simulink library "adi_ad9361_models_org"  (Simulink 10.0)
settings: Solver=VariableStepAuto  StartTime=0.0  StopTime=10.0  RelTol=1e-3
undefined symbols (not defined in the file): ad9361_preload, D, dBval, DCLeak_Matrix, designMultirateFIR, errordlg, fuzz_val, GainImb_Matrix, IP2_Matrix, IP3_Matrix, magnitude
libraries: simrfV2elements x20, simrfV2util1 x10, dsparch4 x8, simrfV2junction1 x8, simulink x8, dspmlti4 x6, ad9361_private x4, simulink_extras x2, dspsigattribs x2, simrfV2sources1 x2, simrfV2_lib x2, dspmathops x2
(part 2 of 2)

== system adi_ad9361_models_org/ad9361_rx/RF_RX/External LNA ==
  ExternalLNA on/off : Inport
  Amplifier : simrfV2elements/Amplifier  classname=amplifier  DataSource=Data file  File=unitygain.s2p  Paramtype=S-parameters  Sparam=[0 0;1 0]  SparamFreq=1e9 Hz  SparamZ0=50  Residues=0  Poles=0  DF={0 0; 1 0}  Source_linear_gain=Available power gain  linear_gain=0 dB  Zin=50  Zout=50  Source_Poly=Even and odd order  Poly_Coeffs=[0 1]  IPType=Output  IP2=inf dBm  IP3=inf dBm  P1dB=inf dBm  Psat=inf dBm  Gcomp=inf dBm  InternalGrounding=on  SourceFreq=Extracted from data source  PlotFreq=[1e9:1e6:3e9] Hz  PlotType=X-Y plane  YParam1=S11  YFormat1=Magnitude (decibels)  YParam2=None  YFormat2=Magnitude (decibels)  YOption=Linear  XOption=Linear  SparamRepresentation=Time domain (rationalfit)  FitTol=-40  FitOpt=Fit individually  AutoImpulseLength=on  ImpulseLength=1e-10 s  MagModeling=off  AddNoise=on  NoiseType=Noise figure  NoiseDist=White  NF=0  MinNF=0  Gopt=0  RN=0  CarrierFreq=0 Hz  NoiseAutoImpulseLength=on  NoiseImpulseLength=1e-10 s  SpecifyOpFreq=off  OpFreq=0 Hz
      settings: SourceProductName=RF Blockset  SourceProductBaseCode=RB
  Bypass : simrfV2junction1/Switch  classname=switch  Ron=0 Ohm  Roff=inf Ohm  Vthres=0.5 V
      settings: SourceProductName=RF Blockset  SourceProductBaseCode=RB
  Invert Control : Subsystem
  LNA on input : simrfV2junction1/Switch  classname=switch  Ron=0 Ohm  Roff=inf Ohm  Vthres=0.5 V
      settings: SourceProductName=RF Blockset  SourceProductBaseCode=RB
  LNA on ouput : simrfV2junction1/Switch  classname=switch  Ron=0 Ohm  Roff=inf Ohm  Vthres=0.5 V
      settings: SourceProductName=RF Blockset  SourceProductBaseCode=RB
  in : PMIOPort  Side=Left
  out : PMIOPort  Port=2  Side=Right
  wires:
  Invert Control/1(Out) -> Bypass/1
  ExternalLNA on/off/1 -> Invert Control/1(In), LNA on input/1, LNA on ouput/1
  connections:
  Amplifier/RConn1 -- LNA on ouput/LConn1
  Amplifier/LConn1 -- LNA on input/RConn1
  in/RConn1 -- Bypass/LConn1 -- LNA on input/LConn1
  LNA on ouput/RConn1 -- out/RConn1 -- Bypass/RConn1

== system adi_ad9361_models_org/ad9361_rx/RF_RX/RF Non Idealities ==
  LPF : Inport
  TIA : Inport  Port=2
  Demod : Inport  Port=3
  LNA : Inport  Port=4
  DetectChange : Subsystem
  RF Non Idealities : Subsystem
  DCLeakage : Outport  VectorParamsAs1DForOutWhenUnconnected=off
  GainImbalance : Outport  Port=2  VectorParamsAs1DForOutWhenUnconnected=off
  IP2 : Outport  Port=3  VectorParamsAs1DForOutWhenUnconnected=off
  IP3 : Outport  Port=4  VectorParamsAs1DForOutWhenUnconnected=off
  wires:
  DetectChange/1(Trigger) -> RF Non Idealities/Trigger
  RF Non Idealities/4(IP3) -> IP3/1
  RF Non Idealities/3(IP2) -> IP2/1
  RF Non Idealities/2(GainImbalance) -> GainImbalance/1
  RF Non Idealities/1(DCLeakage) -> DCLeakage/1
  LNA/1 -> DetectChange/1(In1), RF Non Idealities/1(LNA)
  Demod/1 -> DetectChange/2(In2), RF Non Idealities/2(Demod)
  LPF/1 -> DetectChange/4(In4), RF Non Idealities/4(LPF)
  TIA/1 -> DetectChange/3(In3), RF Non Idealities/3(TIA)

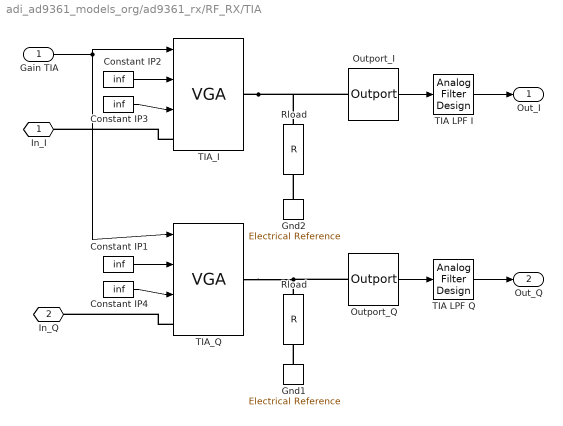
== system adi_ad9361_models_org/ad9361_rx/RF_RX/TIA ==
  Gain TIA : Inport
  " Rload" : simrfV2elements/R  classname=resistor  Resistance=100 Ohm  AddNoise=on
      settings: SourceProductName=RF Blockset  SourceProductBaseCode=RB
  Constant IP{1..4} (4 alike) : Constant  Value=inf
  Gnd1 : simrfV2_lib/Elements/Electrical Reference
      settings: SourceProductName=RF Blockset  SourceProductBaseCode=RB  InternalSimscapePortConfiguration="{\"Bottom\":[],\"Left\":[{\"id\":\"V\",\"label\":\"\",\"type\":\"foundation.rf.circuitenvelope\"}],\"Right\":[],\"Top\":[]}"
  Gnd2 : simrfV2_lib/Elements/Electrical Reference
      settings: SourceProductName=RF Blockset  SourceProductBaseCode=RB  InternalSimscapePortConfiguration="{\"Bottom\":[],\"Left\":[{\"id\":\"V\",\"label\":\"\",\"type\":\"foundation.rf.circuitenvelope\"}],\"Right\":[],\"Top\":[]}"
  Outport_I : simrfV2util1/Outport  SensorType=Ideal voltage  OutputFormat=Real Passband  CarrierFreq=abs(RF-LO) Hz  ZL=Inf  InternalGrounding=on  StepSize=Tstep s  AutoStep=off
      settings: SourceProductName=RF Blockset  SourceProductBaseCode=RB
  Outport_Q : simrfV2util1/Outport  SensorType=Ideal voltage  OutputFormat=Real Passband  CarrierFreq=abs(RF-LO) Hz  ZL=Inf  InternalGrounding=on  StepSize=Tstep s  AutoStep=off
      settings: SourceProductName=RF Blockset  SourceProductBaseCode=RB
  Rload : simrfV2elements/R  classname=resistor  Resistance=100 Ohm  AddNoise=on
      settings: SourceProductName=RF Blockset  SourceProductBaseCode=RB
  TIA LPF I : dsparch4/Analog Filter Design  method=Butterworth  filttype=Lowpass  N=1  Wlo=2.5*ad9361_rx_pars.Fpass*2*pi  Whi=80  Rp=2  Rs=40
  TIA LPF Q : dsparch4/Analog Filter Design  method=Butterworth  filttype=Lowpass  N=1  Wlo=2.5*ad9361_rx_pars.Fpass*2*pi  Whi=80  Rp=2  Rs=40
  TIA_I : simrfV2elements/VGA  classname=vga  Zin=100  Zout=100  IO=Input  InternalGrounding=on
      settings: SourceProductName=RF Blockset  SourceProductBaseCode=RB
  TIA_Q : simrfV2elements/VGA  classname=vga  Zin=100  Zout=100  IO=Input  InternalGrounding=on
      settings: SourceProductName=RF Blockset  SourceProductBaseCode=RB
  In_I : PMIOPort  Side=Left
  In_Q : PMIOPort  Port=2  Side=Left
  Out_I : Outport  VectorParamsAs1DForOutWhenUnconnected=off
  Out_Q : Outport  Port=2  VectorParamsAs1DForOutWhenUnconnected=off
  wires:
  Constant IP4/1 -> TIA_Q/3
  Constant IP1/1 -> TIA_Q/2
  Constant IP3/1 -> TIA_I/3
  Constant IP2/1 -> TIA_I/2
  TIA LPF Q/1 -> Out_Q/1
  TIA LPF I/1 -> Out_I/1
  Gain TIA/1 -> TIA_I/1, TIA_Q/1
  Outport_I/1 -> TIA LPF I/1
  Outport_Q/1 -> TIA LPF Q/1
  connections:
  Gnd1/LConn1 -- " Rload"/RConn1
  Gnd2/LConn1 -- Rload/RConn1
  " Rload"/LConn1 -- TIA_Q/RConn1 -- Outport_Q/LConn1
  TIA_I/RConn1 -- Rload/LConn1 -- Outport_I/LConn1
  TIA_Q/LConn1 -- In_Q/RConn1
  TIA_I/LConn1 -- In_I/RConn1

== system adi_ad9361_models_org/ad9361_rx/Subsystem6/Subsystem1 ==
  Data Type Conversion : DataTypeConversion  OutDataTypeStr=boolean
  Pulse Generator2 : DiscretePulseGenerator  SampleTime=Trf
  START : Outport  VectorParamsAs1DForOutWhenUnconnected=off
  wires:
  Data Type Conversion/1 -> START/1
  Pulse Generator2/1 -> Data Type Conversion/1

== system adi_ad9361_models_org/ad9361_rx/Subsystem6/Wblk5 ==
  Win : Inport
  Sin : Inport  Port=2
  Combinatorial  Logic : CombinatorialLogic  TruthTable=[0; 0; 1; 0]
  Mux : Mux  Inputs=2
  Wout : Outport  VectorParamsAs1DForOutWhenUnconnected=off
  wires:
  Sin/1 -> Mux/2
  Win/1 -> Mux/1
  Combinatorial  Logic/1 -> Wout/1  "wout"
  Mux/1 -> Combinatorial  Logic/1

== system adi_ad9361_models_org/ad9361_rx/Subsystem6/Wblk6 ==
  Win : Inport
  Sin : Inport  Port=2
  Combinatorial  Logic : CombinatorialLogic  TruthTable=[0; 0; 1; 0]
  Mux : Mux  Inputs=2
  Wout : Outport  VectorParamsAs1DForOutWhenUnconnected=off
  wires:
  Sin/1 -> Mux/2
  Win/1 -> Mux/1
  Combinatorial  Logic/1 -> Wout/1  "wout"
  Mux/1 -> Combinatorial  Logic/1

== system adi_ad9361_models_org/ad9361_rx/Subsystem6/Wblk7 ==
  Win : Inport
  Sin : Inport  Port=2
  Combinatorial  Logic : CombinatorialLogic  TruthTable=[0; 0; 1; 0]
  Mux : Mux  Inputs=2
  Wout : Outport  VectorParamsAs1DForOutWhenUnconnected=off
  wires:
  Sin/1 -> Mux/2
  Win/1 -> Mux/1
  Combinatorial  Logic/1 -> Wout/1  "wout"
  Mux/1 -> Combinatorial  Logic/1

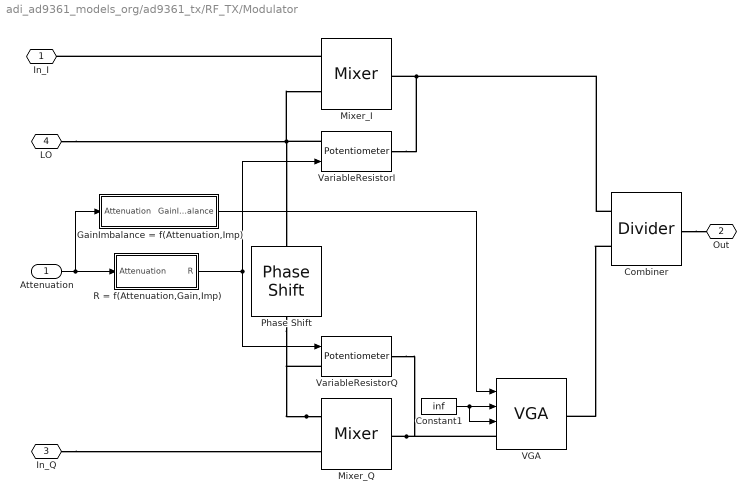
== system adi_ad9361_models_org/ad9361_tx/RF_TX/Modulator ==
  Attenuation : Inport
  "Combiner " : simrfV2junction1/Divider  classname=dividers  DataSource=Network-parameters  NumPorts=3  DeviceCirculator=Circulator clockwise  DeviceDivider=Resistive power divider  DeviceCoupler=Directional coupler  Paramtype=S-parameters  Sparam=[0 0 1; 1 0 0; 0 1 0]  SparamFreq=1e9 Hz  SparamZ0=50  Phase12=0  Phase33=0  Alpha=0  Coupling=0  Directivity=inf  InsertionLoss=inf  ReturnLoss=inf  InternalGrounding=on  SparamRepresentation=Frequency domain  FitOpt=Share all poles  FitTol=-40
      settings: SourceProductName=RF Blockset  SourceProductBaseCode=RB
  Constant1 : Constant  Value=inf
  GainImbalance = f(Attenuation,Imp) : Subsystem
  Mixer_I : simrfV2elements/Mixer  classname=mixer  Source_linear_gain=Available power gain  linear_gain=0 dB  Zin=50  Zout=50  ZLO=inf  Source_Poly=Even and odd order  Poly_Coeffs=[0 1]  IPType=Output  IP2=Inf dBm  IP3=Inf dBm  P1dB=Inf dBm  Psat=Inf dBm  Gcomp=Inf dBm  NF=0  InternalGrounding=on
      settings: SourceProductName=RF Blockset  SourceProductBaseCode=RB
  Mixer_Q : simrfV2elements/Mixer  classname=mixer  Source_linear_gain=Available power gain  linear_gain=0 dB  Zin=50  Zout=50  ZLO=inf  Source_Poly=Even and odd order  Poly_Coeffs=[0 1]  IPType=Output  IP2=Inf dBm  IP3=Inf dBm  P1dB=Inf dBm  Psat=Inf dBm  Gcomp=Inf dBm  NF=0  InternalGrounding=on
      settings: SourceProductName=RF Blockset  SourceProductBaseCode=RB
  Phase Shift : simrfV2elements/Phase Shift  PhaseShift=90 deg  InternalGrounding=on
      settings: SourceProductName=RF Blockset  SourceProductBaseCode=RB
  R = f(Attenuation,Gain,Imp) : Subsystem
  VGA : simrfV2elements/VGA  classname=vga  Zin=50  Zout=50  IO=Input  InternalGrounding=on
      settings: SourceProductName=RF Blockset  SourceProductBaseCode=RB
  VariableResistorI : simrfV2junction1/Potentiometer  classname=potentiometer  Ron=1e-12 Ohm  Roff=1e12 Ohm  CurveType=Linear  PercentLog=20  PercentAnti=80
      settings: SourceProductName=RF Blockset  SourceProductBaseCode=RB
  VariableResistorQ : simrfV2junction1/Potentiometer  classname=potentiometer  Ron=1e-12 Ohm  Roff=1e12 Ohm  CurveType=Linear  PercentLog=20  PercentAnti=80
      settings: SourceProductName=RF Blockset  SourceProductBaseCode=RB
  In_I : PMIOPort  Side=Left
  Out : PMIOPort  Port=2  Side=Right
  In_Q : PMIOPort  Port=3  Side=Left
  LO : PMIOPort  Port=4  Side=Left
  wires:
  Constant1/1 -> VGA/2, VGA/3
  GainImbalance = f(Attenuation,Imp)/1(GainImbalance) -> VGA/1
  Attenuation/1 -> GainImbalance = f(Attenuation,Imp)/1(Attenuation), R = f(Attenuation,Gain,Imp)/1(Attenuation)
  R = f(Attenuation,Gain,Imp)/1(R) -> VariableResistorI/1, VariableResistorQ/1
  connections:
  "Combiner "/LConn2 -- VGA/RConn1
  "Combiner "/RConn1 -- Out/RConn1
  VariableResistorI/RConn1 -- "Combiner "/LConn1 -- Mixer_I/RConn1
  Mixer_Q/RConn1 -- VariableResistorQ/RConn1 -- VGA/LConn1
  In_Q/RConn1 -- Mixer_Q/LConn1
  VariableResistorI/LConn1 -- Mixer_I/LConn2 -- LO/RConn1 -- Phase Shift/LConn1
  Mixer_I/LConn1 -- In_I/RConn1
  Mixer_Q/LConn2 -- VariableResistorQ/LConn1 -- Phase Shift/RConn1

== system adi_ad9361_models_org/ad9361_tx/RF_TX/PA ==
  " Attenuation" : Inport
  Constant : Constant  Value=Gain
  Constant1 : Constant  Value=inf
  Equivalent Noise Floor : simrfV2sources1/Noise  SimulinkInputSignalType=Ideal voltage  NoiseType=White  NoisePSD=4*1.381e-23*290*50*10^(NF/10)  CarrierFreq=fc_RF Hz  AutoImpulseLength=on  ImpulseLength=1e-10 s  InternalGrounding=off
      settings: SourceProductName=RF Blockset  SourceProductBaseCode=RB
  OIP3 = f(Attenuation,OIP3v,Imp) : Subsystem
  VGA : simrfV2elements/VGA  classname=vga  Zin=50  Zout=50  IO=Output  InternalGrounding=on
      settings: SourceProductName=RF Blockset  SourceProductBaseCode=RB
  In : PMIOPort  Side=Left
  Out : PMIOPort  Port=2  Side=Right
  wires:
  Constant1/1 -> VGA/2
  OIP3 = f(Attenuation,OIP3v,Imp)/1(OIP3) -> VGA/3
  " Attenuation"/1 -> OIP3 = f(Attenuation,OIP3v,Imp)/1(Attenuation)
  Constant/1 -> VGA/1
  connections:
  Equivalent Noise Floor/LConn1 -- Out/RConn1
  Equivalent Noise Floor/RConn1 -- VGA/RConn1
  In/RConn1 -- VGA/LConn1

== system adi_ad9361_models_org/ad9361_rx/ADC_RX/ADC_I/Quantizer ==
  u : Inport
  Abs : Abs
  Idealized ADC quantizer : simulink_extras/Additional Discrete/Idealized ADC quantizer  NumberOfConverterBits=3  Vmin=0  Vmax=.8  OutputDataType=double  OutputNegativeValues=off
      settings: SourceProductName=Simulink
  Product : Product
  Saturation : Saturate  UpperLimit=0.41
  Sign : Signum
  y : Outport  VectorParamsAs1DForOutWhenUnconnected=off
  wires:
  Product/1 -> y/1
  Abs/1 -> Saturation/1
  Sign/1 -> Product/2
  Idealized ADC quantizer/1 -> Product/1
  Saturation/1 -> Idealized ADC quantizer/1
  u/1 -> Abs/1, Sign/1

== system adi_ad9361_models_org/ad9361_rx/ADC_RX/ADC_Q/Quantizer ==
  u : Inport
  Abs : Abs
  Idealized ADC quantizer : simulink_extras/Additional Discrete/Idealized ADC quantizer  NumberOfConverterBits=3  Vmin=0  Vmax=.8  OutputDataType=double  OutputNegativeValues=off
      settings: SourceProductName=Simulink
  Product : Product
  Saturation : Saturate  UpperLimit=0.41
  Sign : Signum
  y : Outport  VectorParamsAs1DForOutWhenUnconnected=off
  wires:
  Product/1 -> y/1
  Abs/1 -> Saturation/1
  Sign/1 -> Product/2
  Idealized ADC quantizer/1 -> Product/1
  Saturation/1 -> Idealized ADC quantizer/1
  u/1 -> Abs/1, Sign/1

== system adi_ad9361_models_org/ad9361_rx/RF_RX/Demodulator/R = f(gain, DCleak) ==
  gain : Inport
  DCleak : Inport  Port=2
  Add : Sum  Inputs=--+-+
  Add1 : Sum  Inputs=+-
  Constant1 : Constant  Value=20
  Constant2 : Constant  Value=27
  Constant3 : Constant  Value=3
  Constant4 : Constant  Value=25
  Gain1 : Gain  Gain=(-1)/20
  Gain2 : Gain  Gain=25
  Gain3 : Gain  Gain=1e-12
  expon3 : Math  Operator=10^u  SaturateOnIntegerOverflow=on
  R : Outport  VectorParamsAs1DForOutWhenUnconnected=off
  wires:
  Gain3/1 -> R/1
  expon3/1 -> Gain2/1
  gain/1 -> Add/1
  Add/1 -> Gain1/1
  DCleak/1 -> Add/5
  Constant3/1 -> Add/2
  Constant1/1 -> Add/3
  Constant2/1 -> Add/4
  Gain1/1 -> expon3/1
  Gain2/1 -> Add1/1
  Constant4/1 -> Add1/2
  Add1/1 -> Gain3/1

== system adi_ad9361_models_org/ad9361_rx/RF_RX/Demodulator/y = f(gain, gainImbalance) ==
  gain : Inport
  gainImbalance : Inport  Port=2
  Add2 : Sum
  Constant2 : Constant  Value=2
  Gain4 : Gain  Gain=1/20
  Gain5 : Gain  Gain=1/20
  Gain6 : Gain  Gain=20
  Times1 : Product  Inputs=***
  expon2 : Math  Operator=10^u  SaturateOnIntegerOverflow=on
  expon3 : Math  Operator=10^u  SaturateOnIntegerOverflow=on
  log1 : Math  Operator=log10  SaturateOnIntegerOverflow=on
  y : Outport  VectorParamsAs1DForOutWhenUnconnected=off
  wires:
  Gain6/1 -> y/1
  Constant2/1 -> Times1/3
  gainImbalance/1 -> Gain4/1
  expon3/1 -> Add2/1, Times1/1
  gain/1 -> Gain5/1
  log1/1 -> Gain6/1
  Add2/1 -> log1/1
  Gain4/1 -> expon2/1
  Times1/1 -> Add2/2
  Gain5/1 -> expon3/1
  expon2/1 -> Times1/2

== system adi_ad9361_models_org/ad9361_rx/RF_RX/External LNA/Invert Control ==
  In : Inport
  Data Type Conversion : DataTypeConversion  OutDataTypeStr=boolean
  Data Type Conversion1 : DataTypeConversion  OutDataTypeStr=double
  Logical Operator : Logic  Operator=NOT  AllPortsSameDT=off  OutDataTypeStr=boolean
  Out : Outport  VectorParamsAs1DForOutWhenUnconnected=off
  wires:
  Data Type Conversion1/1 -> Out/1
  Data Type Conversion/1 -> Logical Operator/1
  Logical Operator/1 -> Data Type Conversion1/1
  In/1 -> Data Type Conversion/1

== system adi_ad9361_models_org/ad9361_rx/RF_RX/RF Non Idealities/DetectChange ==
  In1 : Inport
  In2 : Inport  Port=2
  In3 : Inport  Port=3
  In4 : Inport  Port=4
  Detect Change{,1..4} (5 alike) : simulink/Logic and Bit Operations/Detect Change  vinit=0  OutDataTypeStr=boolean
  Logical Operator : Logic  Operator=OR  Inputs=5  AllPortsSameDT=off  OutDataTypeStr=boolean
  Step : Step  Time=2*Tstep  SampleTime=Tstep  VectorParams1D=off  ZeroCross=off
  Trigger : Outport  VectorParamsAs1DForOutWhenUnconnected=off
  wires:
  Step/1 -> Detect Change4/1
  Detect Change4/1 -> Logical Operator/5
  Logical Operator/1 -> Trigger/1
  In1/1 -> Detect Change/1
  Detect Change3/1 -> Logical Operator/1
  In3/1 -> Detect Change2/1
  In2/1 -> Detect Change1/1
  In4/1 -> Detect Change3/1
  Detect Change2/1 -> Logical Operator/2
  Detect Change1/1 -> Logical Operator/3
  Detect Change/1 -> Logical Operator/4

== system adi_ad9361_models_org/ad9361_rx/RF_RX/RF Non Idealities/RF Non Idealities ==
  LNA : Inport
  Demod : Inport  Port=2
  TIA : Inport  Port=3
  LPF : Inport  Port=4
  Trigger : TriggerPort  VariantControl=Variant  PortDimensions=1
  RF NonIdealities : MATLAB Function  TreatAsAtomicUnit=on
      mask init:
      | load ad9361_rx_tables;
  DCLeakage : Outport  VectorParamsAs1DForOutWhenUnconnected=off
  GainImbalance : Outport  Port=2  VectorParamsAs1DForOutWhenUnconnected=off
  IP2 : Outport  Port=3  VectorParamsAs1DForOutWhenUnconnected=off
  IP3 : Outport  Port=4  VectorParamsAs1DForOutWhenUnconnected=off
  wires:
  TIA/1 -> RF NonIdealities/3(TIA)
  Demod/1 -> RF NonIdealities/2(Demod)
  LPF/1 -> RF NonIdealities/4(LPF)
  LNA/1 -> RF NonIdealities/1(LNA)
  RF NonIdealities/4(IP3) -> IP3/1
  RF NonIdealities/3(IP2) -> IP2/1
  RF NonIdealities/2(GainImb) -> GainImbalance/1
  RF NonIdealities/1(Leak) -> DCLeakage/1

== system adi_ad9361_models_org/ad9361_tx/RF_TX/Modulator/GainImbalance = f(Attenuation,Imp) ==
  Attenuation : Inport
  1-D Lookup Table : Lookup_n-D  NumberOfTableDimensions=1  LookupTableObject=''  BreakpointsForDimension1=Attdata  BreakpointsForDimension1FirstPoint=10  BreakpointsForDimension2FirstPoint=10  BreakpointsForDimension1Spacing=12  BreakpointsForDimension2Spacing=12  Table=Gain_imb  ExtrapMethod=Clip  UseLastTableValue=on  InternalRulePriority=Speed  RndMeth=Simplest  InputSameDT=on
  Add : Sum
  Constant : Constant
  Gain : Gain  Gain=20
  Gain1 : Gain  Gain=2
  Power : Math  Operator=10^u  SaturateOnIntegerOverflow=on
  log10 : Math  Operator=log10  SaturateOnIntegerOverflow=on
  GainImbalance : Outport  VectorParamsAs1DForOutWhenUnconnected=off
  wires:
  Gain/1 -> GainImbalance/1
  Add/1 -> log10/1
  Gain1/1 -> Add/1
  Power/1 -> Gain1/1
  Constant/1 -> Add/2
  1-D Lookup Table/1 -> Power/1
  Attenuation/1 -> 1-D Lookup Table/1
  log10/1 -> Gain/1

== system adi_ad9361_models_org/ad9361_tx/RF_TX/Modulator/R = f(Attenuation,Gain,Imp) ==
  Attenuation : Inport
  Add : Sum  Inputs=+-
  Constant : Constant  Value=50
  Gain : Gain  Gain=50*50
  Lookup Table : Lookup_n-D  NumberOfTableDimensions=1  LookupTableObject=''  BreakpointsForDimension1=Attdata  BreakpointsForDimension1FirstPoint=10  BreakpointsForDimension2FirstPoint=10  BreakpointsForDimension1Spacing=12  BreakpointsForDimension2Spacing=12  Table=-LO_leak  ExtrapMethod=Clip  UseLastTableValue=on  InternalRulePriority=Speed  RndMeth=Simplest  InputSameDT=on
  Normalize : Gain  Gain=1e-12
  Sqrt : Sqrt  SaturateOnIntegerOverflow=on
  expon : Math  Operator=10^u  SaturateOnIntegerOverflow=on
  R : Outport  VectorParamsAs1DForOutWhenUnconnected=off
  wires:
  Normalize/1 -> R/1
  expon/1 -> Gain/1
  Add/1 -> Normalize/1
  Gain/1 -> Sqrt/1
  Sqrt/1 -> Add/1
  Attenuation/1 -> Lookup Table/1
  Lookup Table/1 -> expon/1
  Constant/1 -> Add/2

== system adi_ad9361_models_org/ad9361_tx/RF_TX/PA/OIP3 = f(Attenuation,OIP3v,Imp) ==
  Attenuation : Inport
  1-D Lookup Table : Lookup_n-D  NumberOfTableDimensions=1  LookupTableObject=''  BreakpointsForDimension1=Att_ip3  BreakpointsForDimension1FirstPoint=10  BreakpointsForDimension2FirstPoint=10  BreakpointsForDimension1Spacing=12  BreakpointsForDimension2Spacing=12  Table=OIP3v  ExtrapMethod=Clip  UseLastTableValue=on  InternalRulePriority=Speed  RndMeth=Simplest  InputSameDT=on
  OIP3 : Outport  VectorParamsAs1DForOutWhenUnconnected=off
  wires:
  1-D Lookup Table/1 -> OIP3/1
  Attenuation/1 -> 1-D Lookup Table/1

== matlab function ad9361_rx/RF_RX/RF Non Idealities/RF Non Idealities/RF NonIdealities ==
  data: LNA input double; Leak output double; Demod input double; TIA input double; LPF input double; GainImb output double; IP2 output double; IP3 output double; DCLeak_Matrix parameter double; GainImb_Matrix parameter double; IP3_Matrix parameter double; IP2_Matrix parameter double
function [Leak, GainImb, IP2, IP3] =                                    ...
    nonIdealsRF(LNA, Demod, TIA, LPF, DCLeak_Matrix, GainImb_Matrix,    ...
    IP3_Matrix, IP2_Matrix)
%#codegen
coder.extrinsic('griddatan','warning');
IP2 = 200;
IP3 = 200;
Leak = -200;
GainImb = -200;
Leak(:) = griddatan(DCLeak_Matrix(:,1:4), DCLeak_Matrix(:,5),           ...
    [LNA, Demod, TIA, LPF]);
GainImb(:) = griddatan(GainImb_Matrix(:,1:4), GainImb_Matrix(:,5),      ...
    [LNA, Demod, TIA, LPF]);
IP2(:) = griddatan(IP2_Matrix(:,1:4), IP2_Matrix(:,5),[LNA,Demod,TIA,LPF]);
IP3(:) = griddatan(IP3_Matrix(:,1:4), IP3_Matrix(:,5),[LNA,Demod,TIA,LPF]);

if isnan(IP2)
    IP2(:) = griddatan(IP2_Matrix(:,1:4), IP2_Matrix(:,5),              ...
        [LNA, Demod, TIA, LPF],'nearest');
    % Warning('Failed interpolation on IP2');
end
if isnan(IP3)
    IP3(:) = griddatan(IP3_Matrix(:,1:4), IP3_Matrix(:,5),              ...
        [LNA, Demod, TIA, LPF],'nearest');
    % Warning('Failed interpolation on IP3');
end
if isnan(Leak)
    Leak(:) = griddatan(DCLeak_Matrix(:,1:4), DCLeak_Matrix(:,5),       ...
        [LNA, Demod, TIA, LPF],'nearest');
    % Warning('Failed interpolation on DC leakage');
end
if isnan(GainImb)
    GainImb(:) = griddatan(GainImb_Matrix(:,1:4), GainImb_Matrix(:,5),  ...
        [LNA, Demod, TIA, LPF],'nearest');
    % Warning('Failed interpolation on Gain Imbalance');
end

IP2 = 2*(IP2+LNA);

== stateflow chart ad9361_rx/AGC ==
  settings: executeAtInitialization=1
  state InitialState
    entry: gain_index=76;
  state AGC_SEL
  state SlowAttackMode
    state CheckOverloads
    state ResetLMTMeter
    state ResetADCMeter
    state ResetPMeter1
    state ResetPMeter2
    state ResetPMeter3
    state ResetPMeter4
    state DECREASE_GAIN_Inner
      entry:
      gain_index = max(gain_index-AGC_G_dec_slow,0);
    state INCREASE_GAIN_Inner
      entry:
      gain_index = min(gain_index+AGC_G_inc_slow,76);
    state DECREASE_GAIN_Outer
      entry:
      gain_index = max(gain_index-AGC_G_dec_fast,0);
    state INCREASE_GAIN_Outer
      entry:
      gain_index = min(gain_index+AGC_G_inc_fast,76);
    state DECREASE_GAIN_ADC
      exit:
      gain_index = max(gain_index-ADC_G_dec_fast,0);
    state DECREASE_GAIN_LMT
      exit:
      gain_index = max(gain_index-LMT_G_dec_fast,0);
    (default) -> CheckOverloads
    ResetLMTMeter -> CheckOverloads : after(PeakOverLoadWait,sec)
    CheckOverloads -> DECREASE_GAIN_LMT [order 1] : at(N_LMT_H, LMT_H)
    ResetADCMeter -> CheckOverloads : after(PeakOverLoadWait,sec)
    CheckOverloads -> DECREASE_GAIN_ADC [order 2] : at(N_ADC_H, ADC_H)
    ResetPMeter1 -> CheckOverloads : after(SettlingDelay,sec)
    CheckOverloads -> DECREASE_GAIN_Outer [order 3] : [after(C,sec)&&avg_power>PT_HH]
    ResetPMeter2 -> CheckOverloads : after(SettlingDelay,sec)
    CheckOverloads -> DECREASE_GAIN_Inner [order 4] : [after(C,sec)&&avg_power>PT_H]
    ResetPMeter3 -> CheckOverloads : after(SettlingDelay,sec)
    CheckOverloads -> INCREASE_GAIN_Outer [order 5] : [after(C,sec)&&avg_power<PT_LL]
    ResetPMeter4 -> CheckOverloads : after(SettlingDelay,sec)
    CheckOverloads -> INCREASE_GAIN_Inner [order 6] : [after(C,sec)&&avg_power<PT_L]
    DECREASE_GAIN_ADC -> ResetADCMeter : after(C,sec)
    DECREASE_GAIN_Outer -> ResetPMeter1
    DECREASE_GAIN_Inner -> ResetPMeter2
    INCREASE_GAIN_Outer -> ResetPMeter3
    INCREASE_GAIN_Inner -> ResetPMeter4
    DECREASE_GAIN_LMT -> ResetLMTMeter : after(C,sec)
  state ManualGainControl
    state DoNothing
    state CHANGE_GAIN
      entry:
      gain_index = ManualGainIndex;
    (default) -> DoNothing
    CHANGE_GAIN -> DoNothing : after(1e-6,sec)
    DoNothing -> (junction 74) : after(1e-6,sec)
    (junction 74) -> CHANGE_GAIN : [ManualGainIndex>0 && ManualGainIndex<77]
  state FastAttackMode
    state State0
    state DecreaseGainFast
      entry:
      gain_index =max(gain_index-AGC_G_dec_fast,0);
    state State1
      entry:
      Lock = 0;
      count = 0;
    state DecreaseGainSlow
      entry:
      gain_index =max(gain_index-AGC_G_dec_slow,0);
    state Wait
    state State2_measLP
      entry:
      LP = 1;
      during:
      LP = (avg_power<LowPower)*LP;
    state State2A
      entry:
      LP = 1;
      during:
      LP = (avg_power<LowPower)*LP;
    state IncreaseGain
      entry:
      gain_index = min(gain_index+AGC_G_inc_fast,76);
    state State2_setGain
      entry:
      gain_change = min(int8(AGC_lock_level-avg_power), Max_Increase);
      gain_index = min(max(gain_index+gain_change, 0),76);
      gain_begin = gain_index;
    state State3
      entry:
      LP = 1;
      during:
      LP = (avg_power<LowPower)*LP;
    state State4
      entry:
      count = count+1;
      gain_index =max(gain_index-PostLockStepSize,0);
    state State5_measPow
      entry:
      Lock = 1;
      count = 0;
      exit:
      init_power = avg_power;
    state ResetGain
      (default) -> (junction 120)
      (junction 120) -> (junction 121) [order 1] : [GainReset==1]{gain_index=76}
      (junction 120) -> (junction 122) [order 2]
      (junction 122) -> (junction 123) [order 1] : [GainReset==2]{gain_index=min(max(gain_end+GainOffset, 0),76) }
      (junction 122) -> (junction 124) [order 2]
      (junction 124) -> (junction 125) [order 1] : [GainReset==3]{gain_index=gain_begin}
      (junction 124) -> (junction 126) [order 2]
    state PowerMeas_5
      entry:
      PA =avg_power;
      exit:
      gain_end = gain_index;
    state Counter
      entry:
      count = count+1;
    (default) -> State0
    State0 -> State1 : after(AGC_attack_delay*1e-6,sec)
    State2_measLP -> DecreaseGainFast [order 1] : [at(1,LMT_H) || at(1,ADC_H)]
    State1 -> DecreaseGainFast [order 1] : [at(1,LMT_H) || at(1,ADC_H)]
    DecreaseGainFast -> State1 : after(PeakOverLoadWait,sec)
    State2_measLP -> DecreaseGainSlow [order 2] : at(1,ADC_L)
    State1 -> DecreaseGainSlow [order 2] : at(1,ADC_L)
    (junction 81) -> State1
    DecreaseGainSlow -> State1 : after(PeakOverLoadWait,sec)
    (junction 79) -> State1 [order 2]
    State1 -> Wait [order 3] : after(EnergyDetectCount,sec)
    Wait -> State2_measLP : [after(max(SettlingDelay-EnergyDetectCount,0),sec)]
    State2A -> (junction 79) : after(IncrTime, sec)
    (junction 79) -> IncreaseGain [order 1] : [LP && EnableIncrGain]
    IncreaseGain -> State2A : after(DecPowerMeasDuration, sec)
    (junction 82) -> State2A [order 1] : [LP && EnableIncrGain && EnableGainIncAfterLock]/{Lock=0}
    (junction 80) -> State2A [order 1] : [LP && EnableIncrGain]
    State2_measLP -> (junction 80) [order 3] : after(DecPowerMeasDuration, sec)
    (junction 80) -> State2_setGain [order 2]
    State2_setGain -> State3 : {Lock=1;}
    State3 -> State4 [order 1] : [at(1,LMT_H) || at(1,ADC_H)]{Lock = 0}
    State4 -> (junction 81) [order 1] : [count>Overrange]
    ResetGain -> (junction 81)
    (junction 84) -> (junction 81)
    State4 -> State3 [order 2]
    State3 -> (junction 82) [order 2] : after(DecPowerMeasDuration, sec)
    (junction 82) -> State5_measPow [order 2]
    State5_measPow -> PowerMeas_5 : [after(PowerMeasDuration,sec)]
    (junction 83) -> ResetGain [order 1] : [count>2*GainLockExitCount]{Lock=0}
    (junction 83) -> PowerMeas_5 [order 2] : [after(FIR_Ts,sec)]
    Counter -> (junction 83)
    PowerMeas_5 -> PowerMeas_5 [order 2] : [after(PowerMeasDuration,sec)]
    PowerMeas_5 -> Counter [order 4] : [(init_power-PA)>EnergyLost]
    PowerMeas_5 -> (junction 84) [order 1] : [at(1,LMT_H) || at(1,ADC_H)]{Lock=0}
    PowerMeas_5 -> (junction 84) [order 3] : [(PA-init_power)>StrongerSignalThreshold]
  (default) -> InitialState
  InitialState -> AGC_SEL : after(T*1e-6,sec)
  FastAttackMode -> AGC_SEL : [mode!=2]
  AGC_SEL -> SlowAttackMode [order 3] : [mode==0]
  SlowAttackMode -> AGC_SEL : [mode!=0]
  AGC_SEL -> FastAttackMode [order 2] : [mode==2]
  AGC_SEL -> ManualGainControl [order 1] : [mode==1]
  ManualGainControl -> AGC_SEL : [mode!=1]
  data: mode input double; N_LMT_H parameter double; N_ADC_H parameter double; C parameter double; ADC_G_dec_fast parameter double; AGC_G_inc_fast parameter double; AGC_G_inc_slow parameter double; LMT_G_dec_fast parameter double; AGC_G_dec_fast parameter double; AGC_G_dec_slow parameter double; avg_power input double; ManualGainIndex parameter double; AGC_attack_delay parameter double; EnergyDetectCount parameter double; EnableIncrGain parameter double; IncrTime parameter double; FIR_Ts parameter double; T parameter double; AGC_lock_level parameter double; EnableGainIncAfterLock parameter double; Max_Increase parameter double; gain_change local double; Overrange parameter double; PostLockStepSize parameter double; count local double; Lock local double; EnergyLost parameter double; GainLockExitCount parameter double; init_power local double; LowPower parameter double; PowerMeasDuration parameter double; LP local double; PA local double; PeakOverLoadWait parameter double; GainOffset parameter double; StrongerSignalThreshold parameter double; gain_begin local double; GainReset parameter double; PT_H parameter double; PT_HH parameter double; PT_L parameter double; PT_LL parameter double; SettlingDelay parameter double; gain_index output double; DecPowerMeasDuration parameter double; gain_end local double
  events: ADC_H input EITHER_EDGE_EVENT; ADC_L input EITHER_EDGE_EVENT; LMT_L input EITHER_EDGE_EVENT; LMT_H input EITHER_EDGE_EVENT; event input EITHER_EDGE_EVENT
